simulink model "chap5_4sim"  (Simulink 7.7)
settings: Solver=ode45  StartTime=0.0  StopTime=10  FixedStep=0.00000010  RelTol=1e-3
settings Model: Creator=ljk  LastModifiedBy=ljk  ExtModeTrigMode=oneshot  ExtModeArmWhenConnect=off
settings DataIOCC: LimitDataPoints=off  SignalLoggingName=sigsOut
settings OptimizationCC: BooleanDataType=off
settings DebuggingCC: SaveWithParameterizedLinksMsg=none  SignalResolutionControl=TryResolveAllWithWarning  SolverPrmCheckMsg=none  MultiTaskDSMMsg=warning  MultiTaskCondExecSysMsg=none  StrictBusMsg=None
settings HardwareCC: TargetUnknown=on
settings RTWCC: IncludeERTFirstTime=on
settings CodeAppCC: CustomSymbolStrType=$N$R$M_T

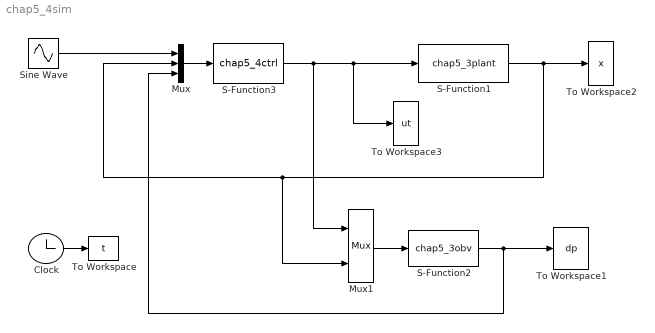
== system chap5_4sim ==
  Clock : Clock
  Mux : Mux  Inputs=3
  Mux1 : Mux  Inputs=2
  S-Function1 : S-Function  FunctionName=chap5_3plant  EnableBusSupport=off
  S-Function2 : S-Function  FunctionName=chap5_3obv  EnableBusSupport=off
  S-Function3 : S-Function  FunctionName=chap5_4ctrl  EnableBusSupport=off
  Sine Wave : Sin  SampleTime=0
  To Workspace : ToWorkspace  VariableName=t  SampleTime=-1  SaveFormat=Array
  To Workspace1 : ToWorkspace  VariableName=dp  SampleTime=-1  SaveFormat=Array
  To Workspace2 : ToWorkspace  VariableName=x  SampleTime=-1  SaveFormat=Array
  To Workspace3 : ToWorkspace  VariableName=ut  SampleTime=-1  SaveFormat=Array
  wires:
  Clock/1 -> To Workspace/1
  Mux1/1 -> S-Function2/1
  S-Function2/1 -> To Workspace1/1, Mux/3
  S-Function1/1 -> To Workspace2/1, Mux1/2, Mux/2
  S-Function3/1 -> Mux1/1, S-Function1/1, To Workspace3/1
  Mux/1 -> S-Function3/1
  Sine Wave/1 -> Mux/1
